simulink model "RocketSimulation_sim"  (R2026a)
settings: Solver=FixedStepAuto  StopTime=tf  FixedStep=dt
undefined symbols (not defined in the file): A, Cd, dt, F2, g, I, Ki, Kp, L, M, p, T

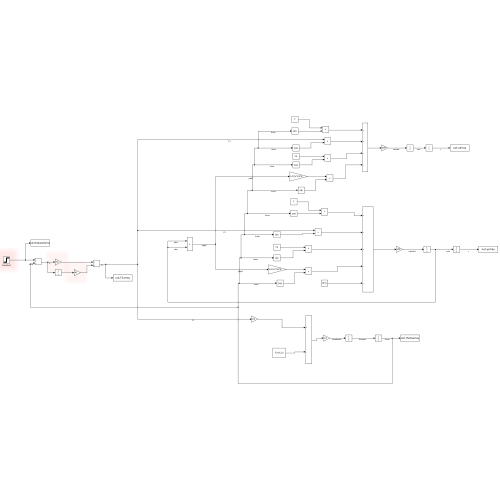
[thumbnail: Simulink's stored preview of the top-level diagram]
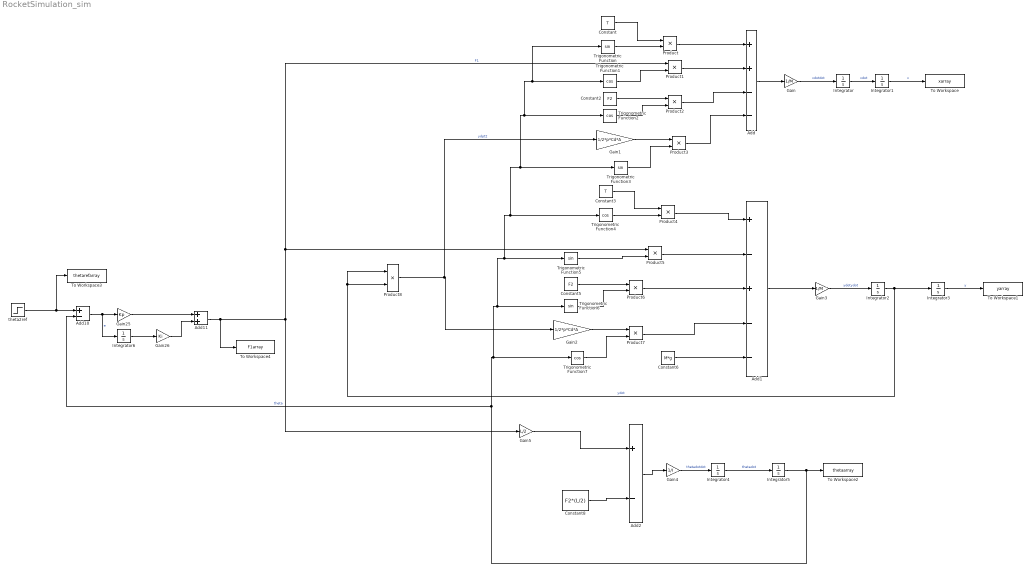
== system RocketSimulation_sim ==
  Add : Sum  Inputs=++--
  Add1 : Sum  Inputs=+-+--
  Add10 : Sum  Inputs=+-
  Add11 : Sum
  Add2 : Sum  Inputs=+-
  Constant : Constant  Value=T
  Constant2 : Constant  Value=F2
  Constant3 : Constant  Value=T
  Constant5 : Constant  Value=F2
  Constant6 : Constant  Value=M*g
  Constant8 : Constant  Value=F2*(L/2)
  Gain : Gain  Gain=1/M
  Gain1 : Gain  Gain=1/2*p*Cd*A
  Gain2 : Gain  Gain=1/2*p*Cd*A
  Gain25 : Gain  Gain=Kp
  Gain26 : Gain  Gain=Ki
  Gain3 : Gain  Gain=1/M
  Gain4 : Gain  Gain=1/I
  Gain5 : Gain  Gain=L/2
  Integrator{,1..6} (7 alike) : Integrator
  Product{,1..8} (9 alike) : Product
  To Workspace : ToWorkspace  VariableName=xarray  SampleTime=-1
  To Workspace1 : ToWorkspace  VariableName=yarray  SampleTime=-1
  To Workspace2 : ToWorkspace  VariableName=thetaarray  SampleTime=-1
  To Workspace3 : ToWorkspace  VariableName=thetarefarray  SampleTime=-1
  To Workspace4 : ToWorkspace  VariableName=F1array  SampleTime=-1
  Trigonometric Function{,3,5..6} (4 alike) : Trigonometry
  Trigonometric Function{1..2,4,7} (4 alike) : Trigonometry  Operator=cos
  theta2ref : Step  Time=dt  FinalValue=thetaref  SampleTime=0
  wires:
  Add/1 -> Gain/1
  Gain/1 -> Integrator/1  "xdotdot"
  Integrator/1 -> Integrator1/1  "xdot"
  Integrator1/1 -> To Workspace/1  "x"
  Product/1 -> Add/1
  Constant/1 -> Product/1
  Trigonometric Function/1 -> Product/2
  Trigonometric Function1/1 -> Product1/2
  Product1/1 -> Add/2
  Constant2/1 -> Product2/1
  Trigonometric Function2/1 -> Product2/2
  Product2/1 -> Add/3
  Gain1/1 -> Product3/1
  Trigonometric Function3/1 -> Product3/2
  Product3/1 -> Add/4
  Constant3/1 -> Product4/1
  Product4/1 -> Add1/1
  Trigonometric Function4/1 -> Product4/2
  Trigonometric Function5/1 -> Product5/2
  Product5/1 -> Add1/2
  Constant5/1 -> Product6/1
  Trigonometric Function6/1 -> Product6/2
  Product6/1 -> Add1/3
  Trigonometric Function7/1 -> Product7/2
  Product7/1 -> Add1/4
  Gain2/1 -> Product7/1
  Constant6/1 -> Add1/5
  Add1/1 -> Gain3/1
  Gain3/1 -> Integrator2/1  "ydotydot"
  Integrator2/1 -> Integrator3/1, Product8/1, Product8/2  "ydot"
  Integrator3/1 -> To Workspace1/1  "y"
  Gain5/1 -> Add2/1
  Constant8/1 -> Add2/2
  Add2/1 -> Gain4/1
  Integrator4/1 -> Integrator5/1  "thetadot"
  Gain4/1 -> Integrator4/1  "thetadotdot"
  Product8/1 -> Gain1/1, Gain2/1  "ydpt2"
  Integrator6/1 -> Gain26/1
  theta2ref/1 -> Add10/1, To Workspace3/1
  Gain25/1 -> Add11/1
  Integrator5/1 -> Add10/2, Trigonometric Function/1, Trigonometric Function1/1, Trigonometric Function2/1, Trigonometric Function3/1, Trigonometric Function4/1, Trigonometric Function5/1, Trigonometric Function6/1, Trigonometric Function7/1, To Workspace2/1  "theta"
  Gain26/1 -> Add11/2
  Add10/1 -> Integrator6/1, Gain25/1  "e"
  Add11/1 -> To Workspace4/1, Gain5/1, Product1/1, Product5/1  "F1"
